simulink model "GPS_coord_conversions"  (R2023a)
settings: Solver=VariableStepAuto  StartTime=0.0  StopTime=10.0  RelTol=1e-3
settings Model: Creator=cbeal  LastModifiedBy=cbeal

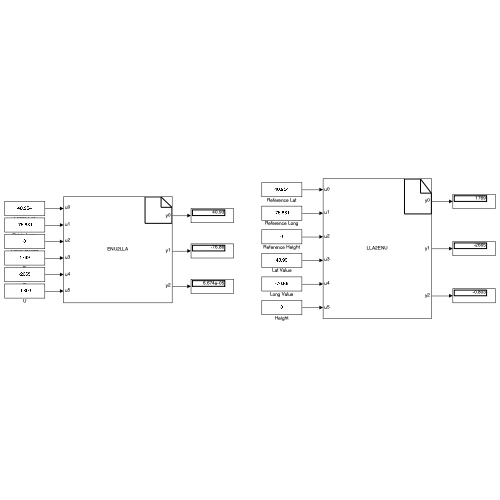
[thumbnail: Simulink's stored preview of the top-level diagram]
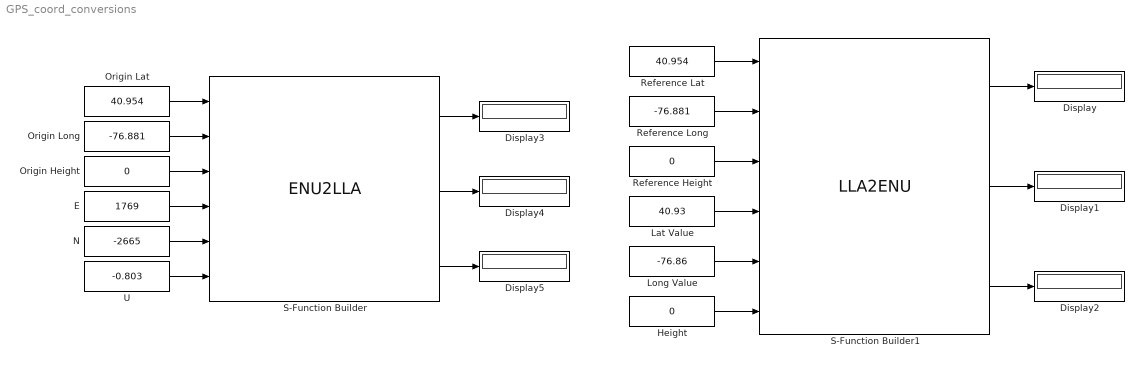
== system GPS_coord_conversions ==
  Display{,1..5} (6 alike) : Display
  E : Constant  Value=1769
  Height : Constant  Value=0
  Lat Value : Constant  Value=40.93
  Long Value : Constant  Value=-76.86
  N : Constant  Value=-2665
  Origin Height : Constant  Value=0
  Origin Lat : Constant  Value=40.954
  Origin Long : Constant  Value=-76.881
  Reference Height : Constant  Value=0
  Reference Lat : Constant  Value=40.954
  Reference Long : Constant  Value=-76.881
  S-Function Builder : S-Function  FunctionName=ENU2LLA  SFunctionModules=ENU2LLA_wrapper.c  SFunctionDeploymentMode=off  EnableBusSupport=off  mask(S-Function Builder){}
      mask help: Simulink:masks:SFunctionBuilder_MD
      mask init:
      | val = [[.9  0.75 0.75 1 1 .9 .9 1]',[1 1 0.75 0.75 .9 .9 1 .9]'];try , sys = get_param(gcb,'SfunBuilderFcnName');if isempty(sys), sys = get_param(gcb,'FunctionName'); end,catch, sys = get_param(gcb,'FunctionName'); end
      settings: CopyFcn=set_param(gcbh,'LinkStatus','none')  OpenFcn=sfunctionwizard(gcbh)
      mask Display:
      | plot(val(:,1),val(:,2))
      | disp(sys)
      | port_label('input',1,'u0')
      | port_label('input',2,'u1')
      | port_label('input',3,'u2')
      | port_label('input',4,'u3')
      | port_label('input',5,'u4')
      | port_label('input',6,'u5')
      | port_label('output',1,'y0')
      | port_label('output',2,'y1')
      | port_label('output',3,'y2')
  S-Function Builder1 : S-Function  FunctionName=LLA2ENU  SFunctionModules=LLA2ENU_wrapper.c  SFunctionDeploymentMode=off  EnableBusSupport=off  mask(S-Function Builder){}
      mask help: Simulink:masks:SFunctionBuilder_MD
      mask init: same as GPS_coord_conversions/S-Function Builder
      settings: CopyFcn=set_param(gcbh,'LinkStatus','none')  OpenFcn=sfunctionwizard(gcbh)
      mask Display:
      | plot(val(:,1),val(:,2))
      | disp(sys)
      | port_label('input',1,'u0')
      | port_label('input',2,'u1')
      | port_label('input',3,'u2')
      | port_label('input',4,'u3')
      | port_label('input',5,'u4')
      | port_label('input',6,'u5')
      | port_label('output',1,'y0')
      | port_label('output',2,'y1')
      | port_label('output',3,'y2')
  U : Constant  Value=-0.803
  wires:
  Origin Lat/1 -> S-Function Builder/1
  Origin Long/1 -> S-Function Builder/2
  Origin Height/1 -> S-Function Builder/3
  E/1 -> S-Function Builder/4
  N/1 -> S-Function Builder/5
  U/1 -> S-Function Builder/6
  S-Function Builder1/1 -> Display/1
  S-Function Builder1/2 -> Display1/1
  S-Function Builder1/3 -> Display2/1
  Reference Lat/1 -> S-Function Builder1/1
  Reference Long/1 -> S-Function Builder1/2
  Reference Height/1 -> S-Function Builder1/3
  Lat Value/1 -> S-Function Builder1/4
  Long Value/1 -> S-Function Builder1/5
  Height/1 -> S-Function Builder1/6
  S-Function Builder/1 -> Display3/1
  S-Function Builder/2 -> Display4/1
  S-Function Builder/3 -> Display5/1
